simulink model "simulation_MRAC"  (R2025b)
settings: Solver=ode1be  StartTime=0.0  StopTime=500  FixedStep=0.001  RelTol=1e-3
values from neighbouring files (symbols this model uses):
  A = -1    [Lyap_matrix.m]
  A_m = -1    [Lyap_matrix.m]
  B = 0.5    [Lyap_matrix.m]
  B_m = 1    [Lyap_matrix.m]
  C = 1    [Lyap_matrix.m]
  D = 0    [Lyap_matrix.m]
settings Model: Creator=drbha  LastModifiedBy=drbha

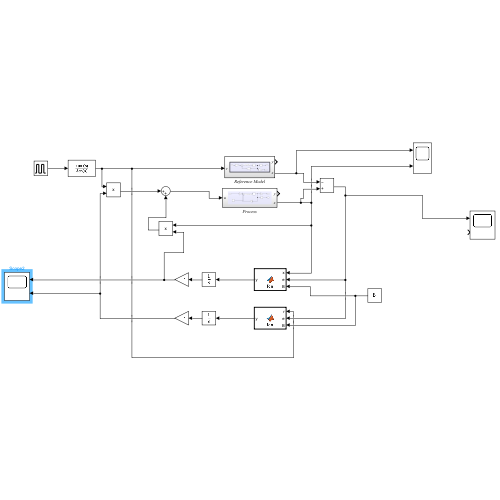
[thumbnail: Simulink's stored preview of the top-level diagram]
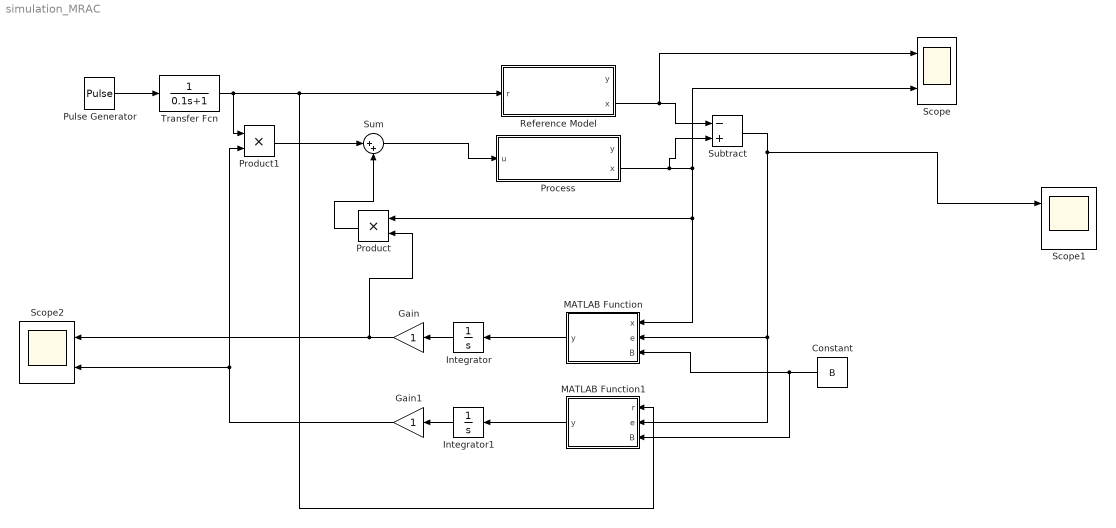
== system simulation_MRAC ==
  Constant : Constant  Value=B
  Gain : Gain
  Gain1 : Gain
  Integrator : Integrator
  Integrator1 : Integrator
  MATLAB Function : MATLAB Function  TreatAsAtomicUnit=on
  MATLAB Function1 : MATLAB Function  TreatAsAtomicUnit=on
  Process : Subsystem
  Product : Product
  Product1 : Product
  Pulse Generator : DiscretePulseGenerator  PulseType=Time based  Period=25  PulseWidth=50
  Reference Model : Subsystem
  Scope : Scope  NumInputPorts=2
      settings: ActiveDisplayYMinimum=-0.13374751121704287  ActiveDisplayYMaximum=1.2037276009533862
  Scope1 : Scope  NumInputPorts=2
      settings: ActiveDisplayYMinimum=-0.90995340165672234  ActiveDisplayYMaximum=0.873695940366499
  Scope2 : Scope  NumInputPorts=2
      settings: ActiveDisplayYMinimum=-2.938777719570826  ActiveDisplayYMaximum=4.2607744567599939  DataLoggingVariableName=ScopeData2
  Subtract : Sum  Inputs=-+
  Sum : Sum  Inputs=|++
  Transfer Fcn : TransferFcn  Denominator=[0.1 1]
  wires:
  Sum/1 -> Process/1(u)
  Pulse Generator/1 -> Transfer Fcn/1
  Subtract/1 -> MATLAB Function1/2(e), MATLAB Function/2(e), Scope1/1
  Reference Model/2(x) -> Scope/1, Subtract/1
  Process/2(x) -> MATLAB Function/1(x), Product/1, Scope/2, Subtract/2
  Transfer Fcn/1 -> Product1/1, Reference Model/1(r), MATLAB Function1/1(r)
  Constant/1 -> MATLAB Function1/3(B), MATLAB Function/3(B)
  MATLAB Function/1(y) -> Integrator/1
  MATLAB Function1/1(y) -> Integrator1/1
  Integrator/1 -> Gain/1
  Integrator1/1 -> Gain1/1
  Gain/1 -> Scope2/1, Product/2
  Product1/1 -> Sum/1
  Gain1/1 -> Scope2/2, Product1/2
  Product/1 -> Sum/2

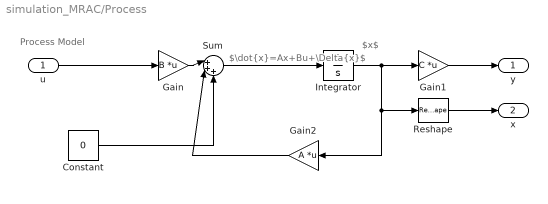
== system simulation_MRAC/Process ==
  note: $\dot{x}=Ax+Bu+\Delta{x}$
  note: Process Model
  note: $x$
  u : Inport
  Constant : Constant  Value=0
  Gain : Gain  Gain=B  Multiplication=Matrix(K*u)
  Gain1 : Gain  Gain=C  Multiplication=Matrix(K*u)
  Gain2 : Gain  Gain=A  Multiplication=Matrix(K*u)
  Integrator : Integrator
  Reshape : Reshape  OutputDimensionality=Column vector (2-D)
  Sum : Sum  Inputs=|+++
  y : Outport
  x : Outport  Port=2
  wires:
  Integrator/1 -> Gain2/1, Reshape/1, Gain1/1
  Sum/1 -> Integrator/1
  Gain1/1 -> y/1
  u/1 -> Gain/1
  Gain2/1 -> Sum/2
  Gain/1 -> Sum/1
  Constant/1 -> Sum/3
  Reshape/1 -> x/1

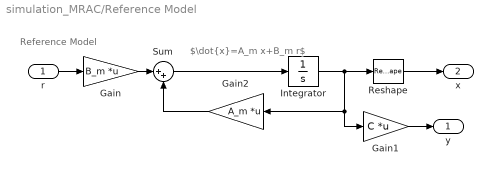
== system simulation_MRAC/Reference Model ==
  note: Reference Model
  note: $\dot{x}=A_m x+B_m r$
  r : Inport
  Gain : Gain  Gain=B_m  Multiplication=Matrix(K*u)
  Gain1 : Gain  Gain=C  Multiplication=Matrix(K*u)
  Gain2 : Gain  Gain=A_m  Multiplication=Matrix(K*u)
  Integrator : Integrator
  Reshape : Reshape  OutputDimensionality=Column vector (2-D)
  Sum : Sum  Inputs=|++
  y : Outport
  x : Outport  Port=2
  wires:
  r/1 -> Gain/1
  Gain/1 -> Sum/1
  Gain2/1 -> Sum/2
  Sum/1 -> Integrator/1
  Gain1/1 -> y/1
  Integrator/1 -> Gain1/1, Gain2/1, Reshape/1
  Reshape/1 -> x/1

== matlab function simulation_MRAC/MATLAB Function ==
  data: x input; y output; e input; B input
function y = fcn(x, e, B)

y = -e*B*x;

== matlab function simulation_MRAC/MATLAB Function1 ==
  data: r input; e input; B input; y output
function y = fcn(r, e, B)

y = -e*B*r;
